simulink model "Lame_sans_graphique"  (R2019b)
settings: Solver=VariableStepAuto  StartTime=0  StopTime=5  FixedStep=0.1  RelTol=1e-3
model workspace (MAT data in the model file):
  F = [0 0 0 0 0 0 0 0 0 0 0 0 0 0 0 0 0 0 0 0 0]
  K = 1
  a1 = 0.000261007117673
  b1 = 0.618793924538
  c1 = 77.6367098126
  coeffs = [11319432.2907 569821497 46409.5443403 1.75479262565e-09]
  dt = 2e-05
  dx = 0.0133333333333
  nx = 21
  w = [0 0 0 0 0 0 0 0 0 0 0 0 0 0 0 0 0 0 0 0 0]
  w_init = [1 2 3 4 5 6 7 8 9 10 11 12 13 14 15 16 17 18 19 20 21]
  w_new = [0 0 0 0 0 0 0 0 0 0 0 0 0 0 0 0 0 0 0 0 0]
  w_old = [0 0 0 0 0 0 0 0 0 0 0 0 0 0 0 0 0 0 0 0 0]
settings Model: Creator=antoi  LastModifiedBy=SAGOU26
settings DebuggingCC: UnderSpecifiedDimensionMsg=warning

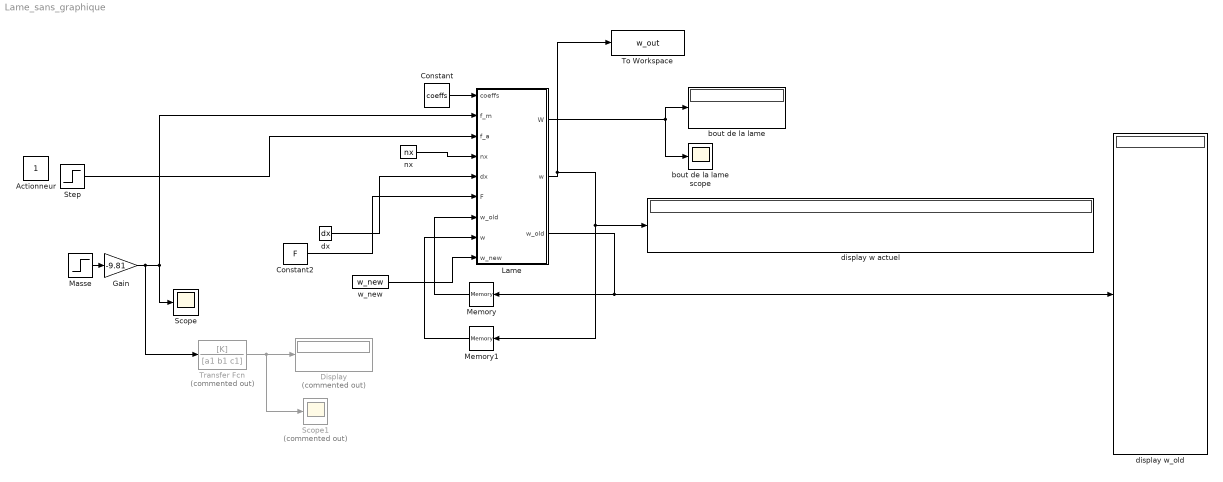
== system Lame_sans_graphique ==
  Actionneur : Constant  SampleTime=dt
  Constant : Constant  Value=coeffs  SampleTime=dt
  Constant2 : Constant  Value=F  SampleTime=dt
  Display : Display  Commented=on
  Gain : Gain  Gain=-9.81
  Lame : MATLAB Function  TreatAsAtomicUnit=on
  Masse : Step  Time=0.5  After=0  SampleTime=dt
  Memory : Memory  InitialCondition=zeros(1,nx)
  Memory1 : Memory  InitialCondition=zeros(1,nx)
  Scope : Scope
  Scope1 : Scope  Commented=on
  Step : Step  Time=0.5  SampleTime=dt
  To Workspace : ToWorkspace  VariableName=w_out  SaveFormat=Timeseries  SampleTime=-1
  Transfer Fcn : TransferFcn  Commented=on  Numerator=[K]  Denominator=[a1 b1 c1]
  bout de la lame : Display
  bout de la lame scope : Scope
  display w actuel : Display
  display w_old : Display
  dx : Constant  Value=dx  SampleTime=dt
  nx : Constant  Value=nx  SampleTime=dt
  w_new : Constant  Value=w_new  SampleTime=dt
  wires:
  Masse/1 -> Gain/1
  Lame/2(w) -> To Workspace/1, Memory1/1, display w actuel/1
  Lame/3(w_old) -> Memory/1, display w_old/1
  Lame/1(W) -> bout de la lame/1, bout de la lame scope/1
  nx/1 -> Lame/4(nx)
  Memory/1 -> Lame/7("w_old ")
  dx/1 -> Lame/5(dx)
  w_new/1 -> Lame/9(w_new)
  Transfer Fcn/1 -> Scope1/1, Display/1
  Constant/1 -> Lame/1(coeffs)
  Gain/1 -> Transfer Fcn/1, Lame/2(f_m), Scope/1
  Constant2/1 -> Lame/6(F)
  Memory1/1 -> Lame/8("w ")
  Step/1 -> Lame/3(f_a)

== matlab function Lame_sans_graphique/Lame ==
  data: coeffs input; f_m input; W output; f_a input; nx input; dx input; F input; w_old input; w input; w_new input; w output; w_old output
function [W, w, w_old] = fcn(coeffs, f_m, f_a, nx, dx, F, w_old, w, w_new) 
     
    % La force
    F(round(nx/2)) = f_a + f_m;

    for i = 3:nx-2
        
        %Équation différentielle résolue par Sam
        w_new(i) = (-coeffs(1)*(w(i+2)-4*w(i+1)+6*w(i)-4*w(i-1)+w(i-2)) - coeffs(2)*(-2*w(i)+w_old(i)) + coeffs(3)*w(i) + F(i)/dx)*coeffs(4);

        %% Conditions limites 
        w_new(1:2) =0;                                 % Clampé à zero, position et dérivée nulle (le bout de la lame est fixe)
        w_new(end-1) = 2*w_new(end-2)-w_new(end-3);    % Libre au bout, dérivées 2e et 3e nulles
        w_new(end) = 2*w_new(end-1)-w_new(end-2);
       
    end
     
    %% Préparation du prochain tour
    
    w_old = w;
    w = w_new;
    W = w(end);
end
